simulink model "LQR_min_obs"  (R2025b)
settings: Solver=ode45  StartTime=0.0  StopTime=400  RelTol=1e-3
values from neighbouring files (symbols this model uses):
  A = [0 1 0 0;     (m_b*g*r^2)/(I_b*l) 0 (m_b*g*r^2)/(I_b) 0 ;      0 0 0 1;    20 0 (M_r*d*g)/I_r 0 ]    [Copy_of_LQR_ctrl.m]    (also in LQR_ctrl.m = [0 1 0 0;     A1(1,1) 0 A1(1,2) 0;     0 0 0 1;     A1(2,1) ; Rlocus_ctrl.m = [0 1 0 0;     A1(1,1) 0 A1(1,2) 0;     0 0 0 1;     A1(2,1) ; State4.m = [0 1 0 0;     A1(1,1) 0 A1(1,2) 0;     0 0 0 1;     A1(2,1) ; pole_placement_ctrl.m = [0 1 0 0;     A1(1,1) 0 0 0;     0 0 0 1;    A1(2,1) 0 A1(2,)
  A_hat = A_bb - Ke_min*A_ab    [Copy_of_LQR_ctrl.m]    (also in LQR_ctrl.m)
  B = -[0 ; 0; 0 ; ((I_w/R) + (M_w+M_r)*R)/(I_r)]    [Copy_of_LQR_ctrl.m]    (also in LQR_ctrl.m = -[0 ; B1(1); 0 ; B1(2)]; Rlocus_ctrl.m = -[0 ; B1(1); 0 ; B1(2)]; State4.m = -[0 ; B1(1); 0 ; B1(2)]; pole_placement_ctrl.m = -[0 ; B1(1); 0 ; B1(2)])
  B_hat = A_hat*Ke_min + A_ba - Ke_min*A_aa    [Copy_of_LQR_ctrl.m]    (also in LQR_ctrl.m)
  C = [0 0 1 0]    [Copy_of_LQR_ctrl.m]    (also in LQR_ctrl.m; Rlocus_ctrl.m = eye(4); State4.m = eye(4); pole_placement_ctrl.m)
  C_hat = zeros(4, nb)    [Copy_of_LQR_ctrl.m]    (also in LQR_ctrl.m)
  D_hat = zeros(4, na)    [Copy_of_LQR_ctrl.m]    (also in LQR_ctrl.m)
  F_hat = B_b - Ke_min*B_a    [Copy_of_LQR_ctrl.m]    (also in LQR_ctrl.m)
  K = lqr(A, B, Q, R)    [State4.m]    (also in pole_placement_ctrl.m = place(A,B,poles))
  x0 = [0.01, 0, deg2rad(5),0]'    [Copy_of_LQR_ctrl.m]    (also in LQR_ctrl.m; State4.m = x0 - x_ref; pole_placement_ctrl.m = [0.005, 0, deg2rad(0.2),0]')
  x0_omin = [-0.002;0;0]    [Copy_of_LQR_ctrl.m]    (also in LQR_ctrl.m = [-0.02;0;0])
settings Model: Creator=Abhi  LastModifiedBy=Abhi
settings HardwareCC: ProdHWDeviceType=AMD->x86-64 (Windows64)

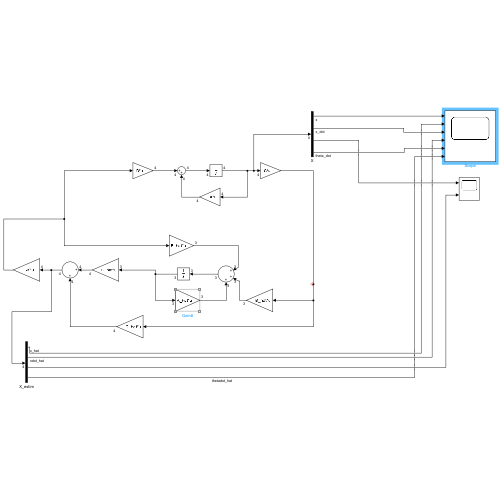
[thumbnail: Simulink's stored preview of the top-level diagram]
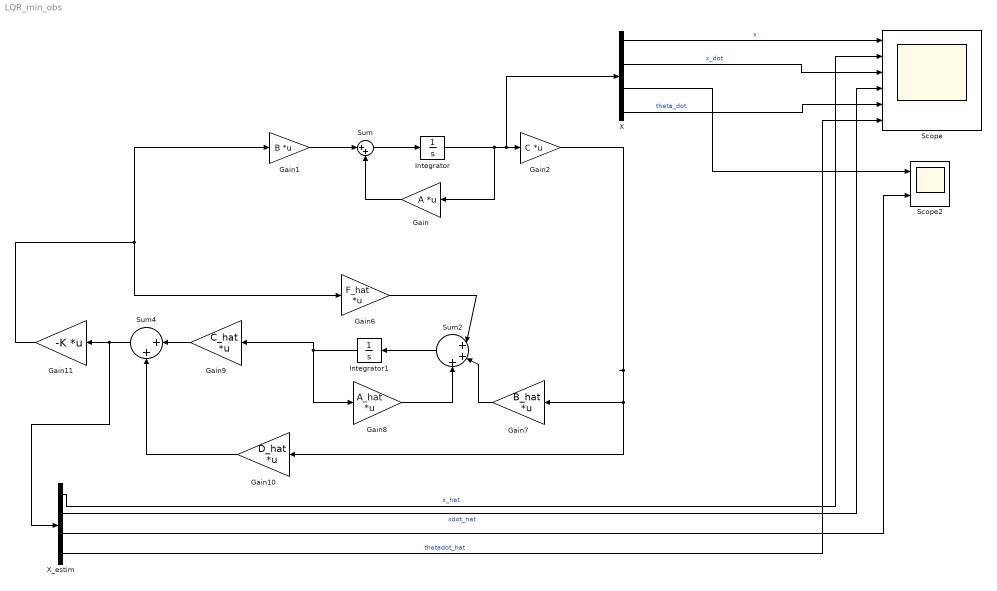
== system LQR_min_obs ==
  Gain : Gain  Gain=A  Multiplication=Matrix(K*u)
  Gain1 : Gain  Gain=B  Multiplication=Matrix(K*u)
  Gain10 : Gain  Gain=D_hat  Multiplication=Matrix(K*u)
  Gain11 : Gain  Gain=-K  Multiplication=Matrix(K*u)
  Gain2 : Gain  Gain=C  Multiplication=Matrix(K*u)
  Gain6 : Gain  Gain=F_hat  Multiplication=Matrix(K*u)
  Gain7 : Gain  Gain=B_hat  Multiplication=Matrix(K*u)
  Gain8 : Gain  Gain=A_hat  Multiplication=Matrix(K*u)
  Gain9 : Gain  Gain=C_hat  Multiplication=Matrix(K*u)
  Integrator : Integrator  InitialCondition=x0
  Integrator1 : Integrator  InitialCondition=x0_omin
  Scope : Scope  NumInputPorts=6
      settings: SampleTime=1e-4  ActiveDisplayYMinimum=-0.039744898058584305  ActiveDisplayYMaximum=0.055584167999339719
  Scope2 : Scope  NumInputPorts=2
      settings: SampleTime=1e-4  ActiveDisplayYMinimum=-0.041102850477065939  ActiveDisplayYMaximum=0.020859803894727538  DataLoggingVariableName=ScopeData2
  Sum : Sum  Inputs=|++
  Sum2 : Sum  Inputs=|+++
  Sum4 : Sum  Inputs=|++
  X : Demux
  X_estim : Demux
  wires:
  Integrator1/1 -> Gain9/1, Gain8/1
  Gain6/1 -> Sum2/1
  Sum4/1 -> X_estim/1, Gain11/1
  Gain/1 -> Sum/2
  Gain8/1 -> Sum2/3
  Sum/1 -> Integrator/1
  Integrator/1 -> X/1, Gain2/1, Gain/1
  Gain7/1 -> Sum2/2
  Gain1/1 -> Sum/1
  Gain11/1 -> Gain1/1, Gain6/1
  Sum2/1 -> Integrator1/1
  Gain10/1 -> Sum4/2
  Gain9/1 -> Sum4/1
  X/1 -> Scope/1  "x"
  X_estim/1 -> Scope/2  "x_hat"
  X/2 -> Scope/3  "x_dot"
  X_estim/2 -> Scope/4  "xdot_hat"
  X/4 -> Scope/5  "theta_dot"
  Gain2/1 -> Gain7/1, Gain10/1
  X_estim/4 -> Scope/6  "thetadot_hat"
  X_estim/3 -> Scope2/2
  X/3 -> Scope2/1
